simulink model "dynamic_plaque_model"  (R2021a)
settings: Solver=FixedStepAuto  StartTime=0.0  StopTime=10.0  RelTol=1e-3
settings Model: Creator=dupa1607  LastModifiedBy=antho
settings SolverCC: AlgebraicLoopSolver=TrustRegion
settings DebuggingCC: SFMachineParentedDataDiag=warning

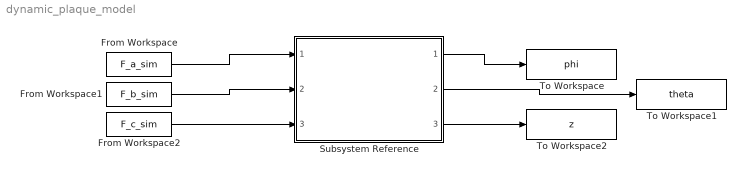
== system dynamic_plaque_model ==
  From Workspace : FromWorkspace  VariableName=F_a_sim
  From Workspace1 : FromWorkspace  VariableName=F_b_sim
  From Workspace2 : FromWorkspace  VariableName=F_c_sim
  Subsystem Reference : Subsystem  ReferencedSubsystem=subsys_dynamic_plaque
  To Workspace : ToWorkspace  VariableName=phi  SaveFormat=Timeseries  SampleTime=-1
  To Workspace1 : ToWorkspace  VariableName=theta  SaveFormat=Timeseries  SampleTime=-1
  To Workspace2 : ToWorkspace  VariableName=z  SaveFormat=Timeseries  SampleTime=-1
  wires:
  From Workspace/1 -> Subsystem Reference/1
  From Workspace1/1 -> Subsystem Reference/2
  From Workspace2/1 -> Subsystem Reference/3
  Subsystem Reference/3 -> To Workspace2/1
  Subsystem Reference/2 -> To Workspace1/1
  Subsystem Reference/1 -> To Workspace/1
